simulink model "KERS_Gesamtmodell"  (Simulink 7.7)
settings: Solver=ode3  StartTime=0.0  StopTime=50.0  FixedStep=TiSample  RelTol=1e-3
model workspace: external: MAT-File ModelWorkspaceGesamtmodell.mat (data not in the file)
values from neighbouring files (symbols this model uses):
  ICnvrSyrmDqMax = 100    [ModelWorkspaceGesamtmodell.mat]
  SpdRtrMecIniVal = 2100    [ModelWorkspaceGesamtmodell.mat]
  SpdRtrMecMax = 2827    [ModelWorkspaceGesamtmodell.mat]
  SpdRtrMecMin = 1131    [ModelWorkspaceGesamtmodell.mat]
  TiSample = 2.5e-06    [ModelWorkspaceGesamtmodell.mat]
  UDcIniVal = 500    [ModelWorkspaceGesamtmodell.mat]
undefined symbols (not defined in the file or in its folder): CDc, CoeffFiltK, CoeffFiltP, CoeffFiltZ, DiscIntNeverNeededParam, JRtr, LSyrmCoilDq_d, LSyrmCoilDq_q, magnitude, NrOfPolePairs, RRepSyrmFeLoss, RSyrmCoilDq
libraries: KERS_SystemModel_lib x29, simulink x6
settings Model: MinMaxOverflowLogging=MinMaxAndOverflow  Creator=johannes.krettek  LastModifiedBy=johannes.krettek
settings DataIOCC: SaveOutput=off  InspectSignalLogs=on  SignalLoggingName=workingLog
settings DebuggingCC: SignalInfNanChecking=warning  UniqueDataStoreMsg=warning

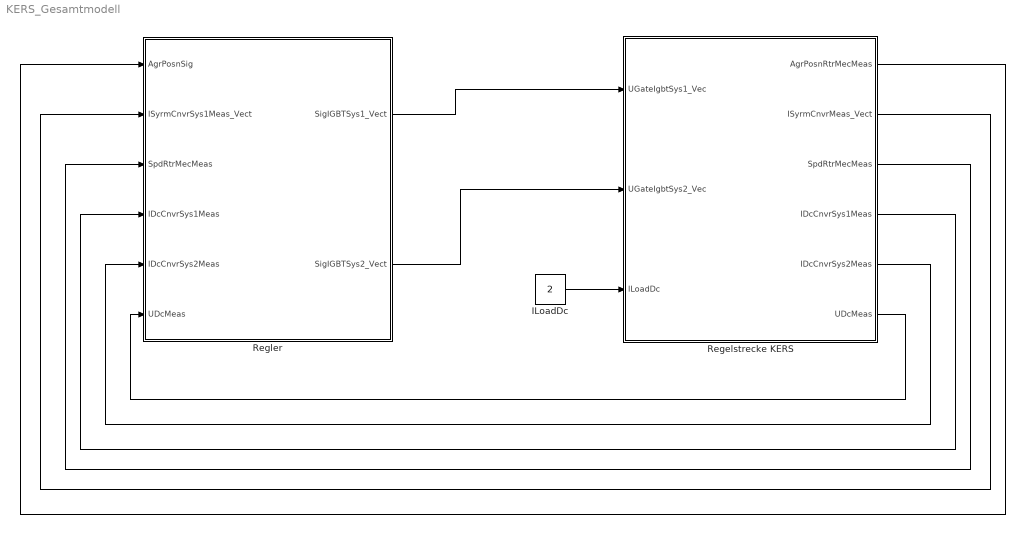
== system KERS_Gesamtmodell ==
  ILoadDc : Constant  Value=2
  Regelstrecke KERS : Subsystem
  Regler : Subsystem
  wires:
  Regler/1(SigIGBTSys1_Vect) -> Regelstrecke KERS/1(UGateIgbtSys1_Vec)
  Regelstrecke KERS/1(AgrPosnRtrMecMeas) -> Regler/1(AgrPosnSig)
  Regelstrecke KERS/2(ISyrmCnvrMeas_Vect) -> Regler/2(ISyrmCnvrSys1Meas_Vect)
  ILoadDc/1 -> Regelstrecke KERS/3(ILoadDc)
  Regler/2(SigIGBTSys2_Vect) -> Regelstrecke KERS/2(UGateIgbtSys2_Vec)
  Regelstrecke KERS/4(IDcCnvrSys1Meas) -> Regler/4(IDcCnvrSys1Meas)
  Regelstrecke KERS/5(IDcCnvrSys2Meas) -> Regler/5(IDcCnvrSys2Meas)
  Regelstrecke KERS/6(UDcMeas) -> Regler/6(UDcMeas)
  Regelstrecke KERS/3(SpdRtrMecMeas) -> Regler/3(SpdRtrMecMeas)

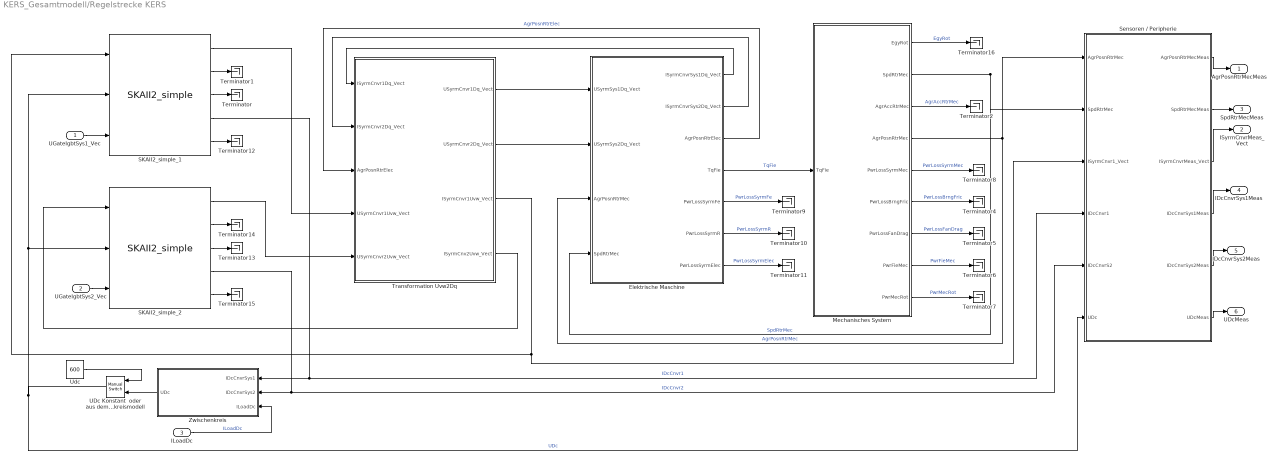
== system KERS_Gesamtmodell/Regelstrecke KERS ==
  UGateIgbtSys1_Vec : Inport  Interpolate=off
  UGateIgbtSys2_Vec : Inport  Port=2  Interpolate=off
  ILoadDc : Inport  Port=3  Interpolate=off
  Elektrische Maschine : Subsystem
  Mechanisches System : Subsystem
  SKAII2_simple_1 : KERS_SystemModel_lib/Leistungselektronik/SKAII2_simple  SystemSampleTime=-1
  SKAII2_simple_2 : KERS_SystemModel_lib/Leistungselektronik/SKAII2_simple  SystemSampleTime=-1
  Sensoren / Peripherie : Subsystem
  Terminator{,1..2,4..16} (16 alike) : Terminator
  Transformation Uvw2Dq : Subsystem
  UDc Konstant  oder aus dem Zwischenkreismodell : simulink/Signal Routing/Manual Switch  SystemSampleTime=-1  sw=0  action=0  varsize=off
  Udc : Constant  Value=600
  Zwischenkreis : Subsystem
  AgrPosnRtrMecMeas : Outport
  ISyrmCnvrMeas_Vect : Outport  Port=2
  SpdRtrMecMeas : Outport  Port=3
  IDcCnvrSys1Meas : Outport  Port=4
  IDcCnvrSys2Meas : Outport  Port=5
  UDcMeas : Outport  Port=6
  wires:
  Mechanisches System/2(SpdRtrMec) -> Elektrische Maschine/4(SpdRtrMec), Sensoren / Peripherie/2(SpdRtrMec)  "SpdRtrMec"
  Mechanisches System/4(AgrPosnRtrMec) -> Elektrische Maschine/3(AgrPosnRtrMec), Sensoren / Peripherie/1(AgrPosnRtrMec)  "AgrPosnRtrMec"
  Elektrische Maschine/4(TqFie) -> Mechanisches System/1(TqFie)  "TqFie"
  UGateIgbtSys1_Vec/1 -> SKAII2_simple_1/3
  Mechanisches System/1(EgyRot) -> Terminator16/1  "EgyRot"
  Mechanisches System/3(AgrAccRtrMec) -> Terminator2/1  "AgrAccRtrMec"
  Elektrische Maschine/5(PwrLossSyrmFe) -> Terminator9/1  "PwrLossSyrmFe"
  Elektrische Maschine/7(PwrLossSyrmElec) -> Terminator11/1  "PwrLossSyrmElec"
  Mechanisches System/6(PwrLossBrngFric) -> Terminator4/1  "PwrLossBrngFric"
  Mechanisches System/7(PwrLossFanDrag) -> Terminator5/1  "PwrLossFanDrag"
  Mechanisches System/9(PwrMecRot) -> Terminator7/1  "PwrMecRot"
  Mechanisches System/5(PwrLossSyrmMec) -> Terminator8/1  "PwrLossSyrmMec"
  Mechanisches System/8(PwrFieMec) -> Terminator6/1  "PwrFieMec"
  Elektrische Maschine/6(PwrLossSyrmR) -> Terminator10/1  "PwrLossSyrmR"
  SKAII2_simple_1/2 -> Terminator1/1
  SKAII2_simple_1/3 -> Terminator/1
  SKAII2_simple_1/5 -> Terminator12/1
  SKAII2_simple_2/2 -> Terminator14/1
  SKAII2_simple_2/3 -> Terminator13/1
  SKAII2_simple_2/5 -> Terminator15/1
  SKAII2_simple_2/4 -> Zwischenkreis/2(IDcCnvrSys2), Sensoren / Peripherie/5(IDcCnvrS2)  "IDcCnvr2"
  UGateIgbtSys2_Vec/1 -> SKAII2_simple_2/3
  Transformation Uvw2Dq/4(ISyrmCnv2Uvw_Vect) -> SKAII2_simple_2/1
  Transformation Uvw2Dq/3(ISyrmCnvr1Uvw_Vect) -> SKAII2_simple_1/1, Sensoren / Peripherie/3(ISyrmCnvr1_Vect)
  Elektrische Maschine/1(ISyrmCnvrSys1Dq_Vect) -> Transformation Uvw2Dq/1(ISyrmCnvr1Dq_Vect)
  Elektrische Maschine/2(ISyrmCnvrSys2Dq_Vect) -> Transformation Uvw2Dq/2(ISyrmCnvr2Dq_Vect)
  Elektrische Maschine/3(AgrPosnRtrElec) -> Transformation Uvw2Dq/3(AgrPosnRtrElec)  "AgrPosnRtrElec"
  Transformation Uvw2Dq/1(USyrmCnvr1Dq_Vect) -> Elektrische Maschine/1(USyrmSys1Dq_Vect)
  Transformation Uvw2Dq/2(USyrmCnvr2Dq_Vect) -> Elektrische Maschine/2(USyrmSys2Dq_Vect)
  SKAII2_simple_1/1 -> Transformation Uvw2Dq/4(USyrmCnvr1Uvw_Vect)
  SKAII2_simple_2/1 -> Transformation Uvw2Dq/5(USyrmCnvr2Uvw_Vect)
  SKAII2_simple_1/4 -> Zwischenkreis/1(IDcCnvrSys1), Sensoren / Peripherie/4(IDcCnvr1)  "IDcCnvr1"
  ILoadDc/1 -> Zwischenkreis/3(ILoadDc)  "ILoadDc"
  Udc/1 -> UDc Konstant  oder aus dem Zwischenkreismodell/1
  Zwischenkreis/1(UDc) -> UDc Konstant  oder aus dem Zwischenkreismodell/2
  UDc Konstant  oder aus dem Zwischenkreismodell/1 -> SKAII2_simple_2/2, SKAII2_simple_1/2, Sensoren / Peripherie/6(UDc)  "UDc"
  Sensoren / Peripherie/3(ISyrmCnvrMeas_Vect) -> ISyrmCnvrMeas_Vect/1
  Sensoren / Peripherie/4(IDcCnvrSys1Meas) -> IDcCnvrSys1Meas/1
  Sensoren / Peripherie/5(IDcCnvrSys2Meas) -> IDcCnvrSys2Meas/1
  Sensoren / Peripherie/1(AgrPosnRtrMecMeas) -> AgrPosnRtrMecMeas/1
  Sensoren / Peripherie/6(UDcMeas) -> UDcMeas/1
  Sensoren / Peripherie/2(SpdRtrMecMeas) -> SpdRtrMecMeas/1

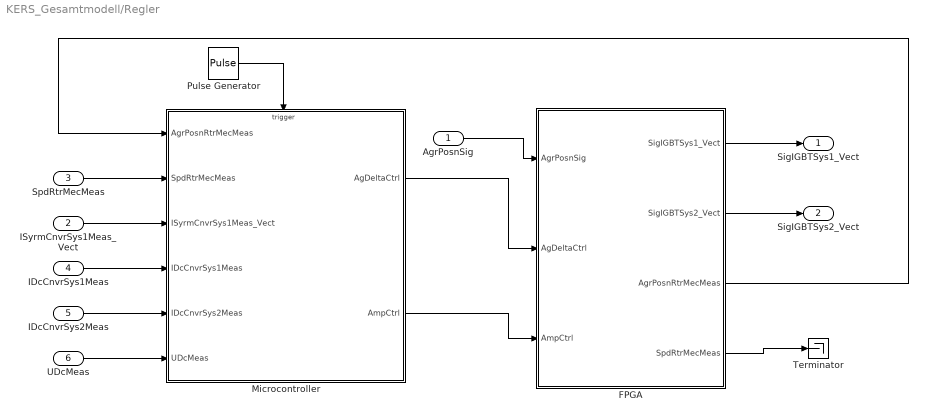
== system KERS_Gesamtmodell/Regler ==
  AgrPosnSig : Inport
  ISyrmCnvrSys1Meas_Vect : Inport  Port=2
  SpdRtrMecMeas : Inport  Port=3
  IDcCnvrSys1Meas : Inport  Port=4
  IDcCnvrSys2Meas : Inport  Port=5
  UDcMeas : Inport  Port=6
  FPGA : Subsystem
  Microcontroller : Subsystem
  Pulse Generator : DiscretePulseGenerator  PulseType=Time based  Period=TiSample*10  PulseWidth=50
  Terminator : Terminator
  SigIGBTSys1_Vect : Outport
  SigIGBTSys2_Vect : Outport  Port=2
  wires:
  FPGA/1(SigIGBTSys1_Vect) -> SigIGBTSys1_Vect/1
  FPGA/2(SigIGBTSys2_Vect) -> SigIGBTSys2_Vect/1
  Microcontroller/1(AgDeltaCtrl) -> FPGA/2(AgDeltaCtrl)
  Microcontroller/2(AmpCtrl) -> FPGA/3(AmpCtrl)
  AgrPosnSig/1 -> FPGA/1(AgrPosnSig)
  FPGA/3(AgrPosnRtrMecMeas) -> Microcontroller/1(AgrPosnRtrMecMeas)
  ISyrmCnvrSys1Meas_Vect/1 -> Microcontroller/3(ISyrmCnvrSys1Meas_Vect)
  IDcCnvrSys1Meas/1 -> Microcontroller/4(IDcCnvrSys1Meas)
  IDcCnvrSys2Meas/1 -> Microcontroller/5(IDcCnvrSys2Meas)
  UDcMeas/1 -> Microcontroller/6(UDcMeas)
  Pulse Generator/1 -> Microcontroller/Trigger
  SpdRtrMecMeas/1 -> Microcontroller/2(SpdRtrMecMeas)
  FPGA/4(SpdRtrMecMeas) -> Terminator/1

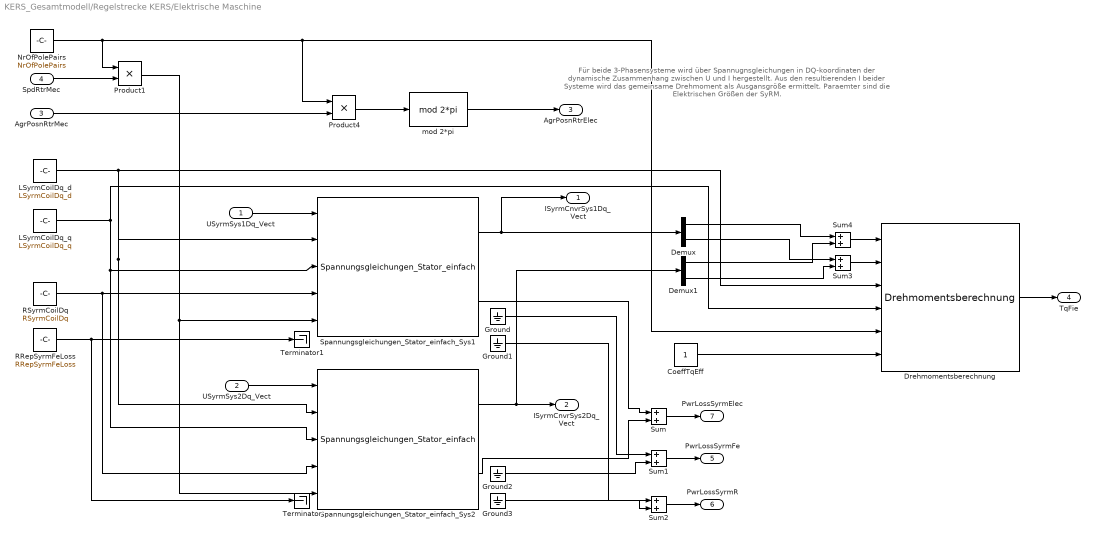
== system KERS_Gesamtmodell/Regelstrecke KERS/Elektrische Maschine ==
  note: Für beide 3-Phasensysteme wird über Spannugnsgleichungen in
      | DQ-koordinaten der dynamische Zusammenhang zwischen U und I
      | hergestellt. Aus den resultierenden I beider Systeme wird das
      | gemeinsame Drehmoment als Ausgansgröße ermittelt.
      | Paraemter sind die Elektrischen Größen der SyRM.
  USyrmSys1Dq_Vect : Inport
  USyrmSys2Dq_Vect : Inport  Port=2
  AgrPosnRtrMec : Inport  Port=3
  SpdRtrMec : Inport  Port=4
  CoeffTqEff : Constant  OutMin=0
  Demux : Demux  Outputs=2
  Demux1 : Demux  Outputs=2
  Drehmomentsberechnung : KERS_SystemModel_lib/Module Stator-Komponenten/Drehmomentsberechnung  SystemSampleTime=-1
  Ground{,1..3} (4 alike) : Ground
  LSyrmCoilDq_d : Constant  Value=LSyrmCoilDq_d  OutMin=0
  LSyrmCoilDq_q : Constant  Value=LSyrmCoilDq_q  OutMin=0
  NrOfPolePairs : Constant  Value=NrOfPolePairs
  Product1 : Product  RndMeth=Zero
  Product4 : Product  RndMeth=Zero
  RRepSyrmFeLoss : Constant  Value=RRepSyrmFeLoss  OutMin=0
  RSyrmCoilDq : Constant  Value=RSyrmCoilDq  OutMin=0
  Spannungsgleichungen_Stator_einfach_Sys1 : KERS_SystemModel_lib/Module Stator-Komponenten/Spannungsgleichungen_Stator_einfach  SystemSampleTime=-1
  Spannungsgleichungen_Stator_einfach_Sys2 : KERS_SystemModel_lib/Module Stator-Komponenten/Spannungsgleichungen_Stator_einfach  SystemSampleTime=-1
  Sum{,1..4} (5 alike) : Sum
  Terminator : Terminator
  Terminator1 : Terminator
  mod 2*pi : KERS_SystemModel_lib/Transformationen/mod 2*pi  SystemSampleTime=-1  tau=2*pi
  ISyrmCnvrSys1Dq_Vect : Outport
  ISyrmCnvrSys2Dq_Vect : Outport  Port=2
  AgrPosnRtrElec : Outport  Port=3
  TqFie : Outport  Port=4
  PwrLossSyrmFe : Outport  Port=5
  PwrLossSyrmR : Outport  Port=6
  PwrLossSyrmElec : Outport  Port=7
  wires:
  Drehmomentsberechnung/1 -> TqFie/1
  LSyrmCoilDq_d/1 -> Drehmomentsberechnung/3, Spannungsgleichungen_Stator_einfach_Sys2/2, Spannungsgleichungen_Stator_einfach_Sys1/2
  LSyrmCoilDq_q/1 -> Drehmomentsberechnung/4, Spannungsgleichungen_Stator_einfach_Sys1/3, Spannungsgleichungen_Stator_einfach_Sys2/3
  NrOfPolePairs/1 -> Product4/1, Drehmomentsberechnung/5, Product1/1
  Product4/1 -> mod 2*pi/1
  Product1/1 -> Spannungsgleichungen_Stator_einfach_Sys2/5, Spannungsgleichungen_Stator_einfach_Sys1/5
  Spannungsgleichungen_Stator_einfach_Sys1/1 -> ISyrmCnvrSys1Dq_Vect/1, Demux/1
  RSyrmCoilDq/1 -> Spannungsgleichungen_Stator_einfach_Sys1/4, Spannungsgleichungen_Stator_einfach_Sys2/4
  AgrPosnRtrMec/1 -> Product4/2
  RRepSyrmFeLoss/1 -> Terminator/1, Terminator1/1
  CoeffTqEff/1 -> Drehmomentsberechnung/6
  mod 2*pi/1 -> AgrPosnRtrElec/1
  Spannungsgleichungen_Stator_einfach_Sys2/1 -> ISyrmCnvrSys2Dq_Vect/1, Demux1/1
  USyrmSys2Dq_Vect/1 -> Spannungsgleichungen_Stator_einfach_Sys2/1
  Sum/1 -> PwrLossSyrmElec/1
  Sum1/1 -> PwrLossSyrmFe/1
  Sum2/1 -> PwrLossSyrmR/1
  Spannungsgleichungen_Stator_einfach_Sys2/2 -> Sum/2
  Ground/1 -> Sum1/1
  Ground2/1 -> Sum1/2
  Ground1/1 -> Sum2/1
  Ground3/1 -> Sum2/2
  Demux/1 -> Sum4/1
  Demux1/1 -> Sum4/2
  Demux/2 -> Sum3/1
  Demux1/2 -> Sum3/2
  Sum4/1 -> Drehmomentsberechnung/1
  Sum3/1 -> Drehmomentsberechnung/2
  Spannungsgleichungen_Stator_einfach_Sys1/2 -> Sum/1
  USyrmSys1Dq_Vect/1 -> Spannungsgleichungen_Stator_einfach_Sys1/1
  SpdRtrMec/1 -> Product1/2

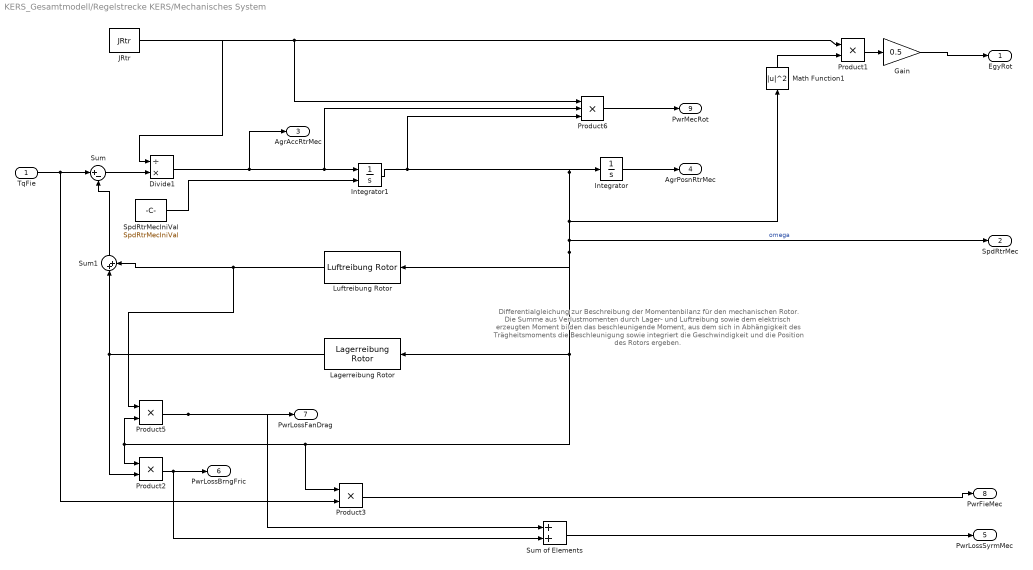
== system KERS_Gesamtmodell/Regelstrecke KERS/Mechanisches System ==
  note: Differentialgleichung zur Beschreibung der Momentenbilanz für den mechanischen Rotor.
      | Die Summe aus Verlustmomenten durch Lager- und Luftreibung sowie dem elektrisch erzeugten
      | Moment bilden das beschleunigende Moment, aus dem sich in Abhängigkeit des Trägheitsmoments
      | die Beschleunigung sowie integriert die Geschwindigkeit und die Position des Rotors ergeben.
  TqFie : Inport
  Divide1 : Product  Inputs=/*
  Gain : Gain  Gain=0.5
  Integrator : Integrator
  Integrator1 : Integrator  InitialConditionSource=external
  JRtr : Constant  Value=JRtr
  Lagerreibung Rotor : KERS_SystemModel_lib/Module Rotor-Komponenten/Lagerreibung Rotor  SystemSampleTime=-1
  Luftreibung Rotor : KERS_SystemModel_lib/Module Rotor-Komponenten/Luftreibung Rotor  SystemSampleTime=-1
  Math Function1 : Math  Operator=magnitude^2  SaturateOnIntegerOverflow=on
  Product{1..3,5} (4 alike) : Product  RndMeth=Zero
  Product6 : Product  Inputs=3  RndMeth=Zero
  SpdRtrMecIniVal : Constant  Value=SpdRtrMecIniVal
  Sum : Sum  Inputs=|+-
  Sum of Elements : Sum
  Sum1 : Sum  Inputs=|++
  EgyRot : Outport
  SpdRtrMec : Outport  Port=2
  AgrAccRtrMec : Outport  Port=3
  AgrPosnRtrMec : Outport  Port=4
  PwrLossSyrmMec : Outport  Port=5
  PwrLossBrngFric : Outport  Port=6
  PwrLossFanDrag : Outport  Port=7
  PwrFieMec : Outport  Port=8
  PwrMecRot : Outport  Port=9
  wires:
  TqFie/1 -> Sum/1, Product3/2
  Sum1/1 -> Sum/2
  Integrator/1 -> AgrPosnRtrMec/1
  Luftreibung Rotor/1 -> Sum1/2, Product5/1
  Lagerreibung Rotor/1 -> Sum1/1, Product2/2
  JRtr/1 -> Divide1/1, Product1/1, Product6/1
  Product1/1 -> Gain/1
  Product2/1 -> PwrLossBrngFric/1, Sum of Elements/2
  Product5/1 -> PwrLossFanDrag/1, Sum of Elements/1
  Product3/1 -> PwrFieMec/1
  Integrator1/1 -> Product5/2, Product2/1, Product3/1, Lagerreibung Rotor/1, Luftreibung Rotor/1, SpdRtrMec/1, Math Function1/1, Integrator/1, Product6/3  "omega"
  Divide1/1 -> AgrAccRtrMec/1, Product6/2, Integrator1/1
  Sum/1 -> Divide1/2
  SpdRtrMecIniVal/1 -> Integrator1/2
  Gain/1 -> EgyRot/1
  Product6/1 -> PwrMecRot/1
  Sum of Elements/1 -> PwrLossSyrmMec/1
  Math Function1/1 -> Product1/2

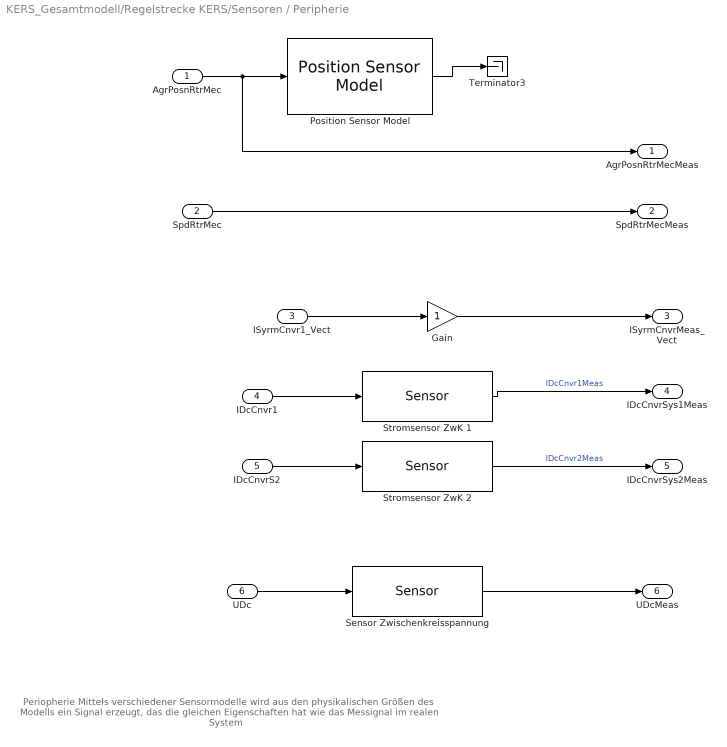
== system KERS_Gesamtmodell/Regelstrecke KERS/Sensoren / Peripherie ==
  note: Periopherie
      | Mittels verschiedener Sensormodelle wird aus den physikalischen Größen
      | des Modells ein Signal erzeugt, das die gleichen Eigenschaften hat wie
      | das Messignal im realen System
  AgrPosnRtrMec : Inport
  SpdRtrMec : Inport  Port=2
  ISyrmCnvr1_Vect : Inport  Port=3
  IDcCnvr1 : Inport  Port=4
  IDcCnvrS2 : Inport  Port=5
  UDc : Inport  Port=6
  Gain : Gain
  Position Sensor Model : KERS_SystemModel_lib/Peripheral Modules/Position Sensor Model  SystemSampleTime=-1  PosnSens1Offset=0.1  PosnSens2Offset=pi  PosnSensWidth=0.2
  Sensor Zwischenkreisspannung : KERS_SystemModel_lib/Peripheral Modules/Sensor  SystemSampleTime=-1
  Stromsensor ZwK 1 : KERS_SystemModel_lib/Peripheral Modules/Sensor  SystemSampleTime=-1
      link override Transport Delay: DelayTime=TiSample
  Stromsensor ZwK 2 : KERS_SystemModel_lib/Peripheral Modules/Sensor  SystemSampleTime=-1
      link override Transport Delay: DelayTime=TiSample
  Terminator3 : Terminator
  AgrPosnRtrMecMeas : Outport
  SpdRtrMecMeas : Outport  Port=2
  ISyrmCnvrMeas_Vect : Outport  Port=3
  IDcCnvrSys1Meas : Outport  Port=4
  IDcCnvrSys2Meas : Outport  Port=5
  UDcMeas : Outport  Port=6
  wires:
  Stromsensor ZwK 1/1 -> IDcCnvrSys1Meas/1  "IDcCnvr1Meas"
  Stromsensor ZwK 2/1 -> IDcCnvrSys2Meas/1  "IDcCnvr2Meas"
  Sensor Zwischenkreisspannung/1 -> UDcMeas/1
  ISyrmCnvr1_Vect/1 -> Gain/1
  AgrPosnRtrMec/1 -> Position Sensor Model/1, AgrPosnRtrMecMeas/1
  UDc/1 -> Sensor Zwischenkreisspannung/1
  IDcCnvr1/1 -> Stromsensor ZwK 1/1
  IDcCnvrS2/1 -> Stromsensor ZwK 2/1
  SpdRtrMec/1 -> SpdRtrMecMeas/1
  Gain/1 -> ISyrmCnvrMeas_Vect/1
  Position Sensor Model/1 -> Terminator3/1

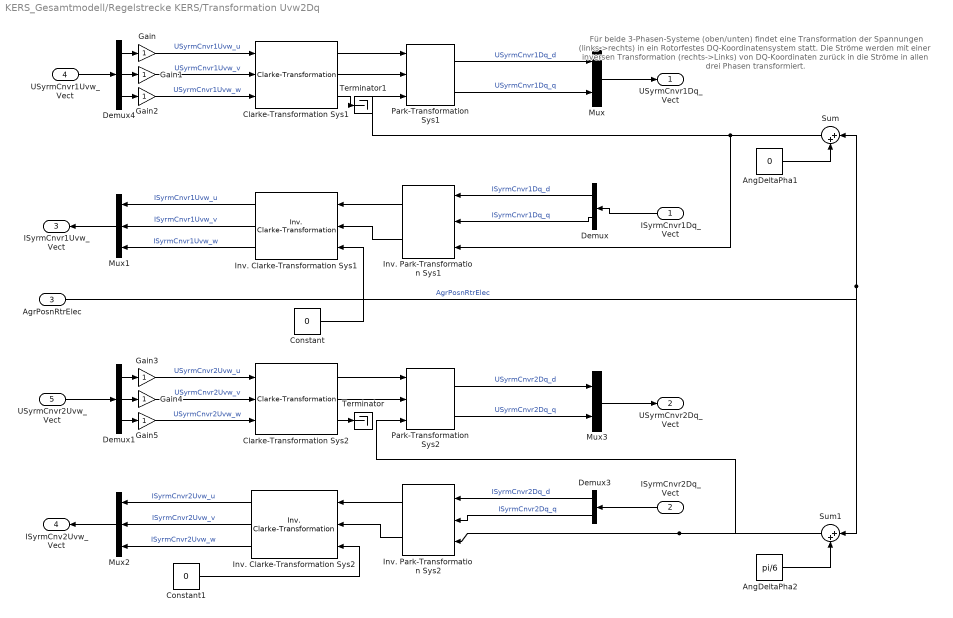
== system KERS_Gesamtmodell/Regelstrecke KERS/Transformation Uvw2Dq ==
  note: Für beide 3-Phasen-Systeme (oben/unten) findet eine Transformation
      | der Spannungen (links->rechts) in ein Rotorfestes DQ-Koordinatensystem statt.
      | Die Ströme werden mit einer inversen Transformation (rechts->Links)
      | von DQ-Koordinaten zurück in die Ströme in allen drei Phasen transformiert.
  ISyrmCnvr1Dq_Vect : Inport
  ISyrmCnvr2Dq_Vect : Inport  Port=2
  AgrPosnRtrElec : Inport  Port=3
  USyrmCnvr1Uvw_Vect : Inport  Port=4
  USyrmCnvr2Uvw_Vect : Inport  Port=5
  AngDeltaPha1 : Constant  Value=0
  AngDeltaPha2 : Constant  Value=pi/6
  Clarke-Transformation Sys1 : KERS_SystemModel_lib/Transformationen/Clarke-Transformation  SystemSampleTime=-1
  Clarke-Transformation Sys2 : KERS_SystemModel_lib/Transformationen/Clarke-Transformation  SystemSampleTime=-1
  Constant : Constant  Value=0
  Constant1 : Constant  Value=0
  Demux : Demux  Outputs=2
  Demux1 : Demux  Outputs=3
  Demux3 : Demux  Outputs=2
  Demux4 : Demux  Outputs=3
  Gain{,1..5} (6 alike) : Gain
  Inv. Clarke-Transformation Sys1 : KERS_SystemModel_lib/Transformationen/Inv. Clarke-Transformation  SystemSampleTime=-1
  Inv. Clarke-Transformation Sys2 : KERS_SystemModel_lib/Transformationen/Inv. Clarke-Transformation  SystemSampleTime=-1
  Inv. Park-Transformation Sys1 : KERS_SystemModel_lib/Transformationen/Inv. Park-Transformation  SystemSampleTime=-1
  Inv. Park-Transformation Sys2 : KERS_SystemModel_lib/Transformationen/Inv. Park-Transformation  SystemSampleTime=-1
  Mux : Mux  Inputs=2
  Mux1 : Mux  Inputs=3
  Mux2 : Mux  Inputs=3
  Mux3 : Mux  Inputs=2
  Park-Transformation Sys1 : KERS_SystemModel_lib/Transformationen/Park-Transformation  SystemSampleTime=-1
  Park-Transformation Sys2 : KERS_SystemModel_lib/Transformationen/Park-Transformation  SystemSampleTime=-1
  Sum : Sum  Inputs=|++
  Sum1 : Sum  Inputs=|++
  Terminator : Terminator
  Terminator1 : Terminator
  USyrmCnvr1Dq_Vect : Outport
  USyrmCnvr2Dq_Vect : Outport  Port=2
  ISyrmCnvr1Uvw_Vect : Outport  Port=3
  ISyrmCnv2Uvw_Vect : Outport  Port=4
  wires:
  Inv. Park-Transformation Sys1/1 -> Inv. Clarke-Transformation Sys1/1
  Inv. Park-Transformation Sys1/2 -> Inv. Clarke-Transformation Sys1/2
  Demux/1 -> Inv. Park-Transformation Sys1/1  "ISyrmCnvr1Dq_d"
  Demux/2 -> Inv. Park-Transformation Sys1/2  "ISyrmCnvr1Dq_q"
  Park-Transformation Sys1/1 -> Mux/1  "USyrmCnvr1Dq_d"
  Park-Transformation Sys1/2 -> Mux/2  "USyrmCnvr1Dq_q"
  Inv. Clarke-Transformation Sys1/1 -> Mux1/1  "ISyrmCnvr1Uvw_u"
  Inv. Clarke-Transformation Sys1/2 -> Mux1/2  "ISyrmCnvr1Uvw_v"
  Inv. Clarke-Transformation Sys1/3 -> Mux1/3  "ISyrmCnvr1Uvw_w"
  ISyrmCnvr1Dq_Vect/1 -> Demux/1
  Mux/1 -> USyrmCnvr1Dq_Vect/1
  Gain/1 -> Clarke-Transformation Sys1/1  "USyrmCnvr1Uvw_u"
  Gain1/1 -> Clarke-Transformation Sys1/2  "USyrmCnvr1Uvw_v"
  Gain2/1 -> Clarke-Transformation Sys1/3  "USyrmCnvr1Uvw_w"
  Gain3/1 -> Clarke-Transformation Sys2/1  "USyrmCnvr2Uvw_u"
  Gain4/1 -> Clarke-Transformation Sys2/2  "USyrmCnvr2Uvw_v"
  Gain5/1 -> Clarke-Transformation Sys2/3  "USyrmCnvr2Uvw_w"
  Clarke-Transformation Sys1/1 -> Park-Transformation Sys1/1
  Clarke-Transformation Sys1/2 -> Park-Transformation Sys1/2
  AgrPosnRtrElec/1 -> Sum/1, Sum1/1  "AgrPosnRtrElec"
  AngDeltaPha1/1 -> Sum/2
  Sum/1 -> Inv. Park-Transformation Sys1/3, Park-Transformation Sys1/3
  AngDeltaPha2/1 -> Sum1/2
  Clarke-Transformation Sys2/1 -> Park-Transformation Sys2/1
  Clarke-Transformation Sys2/2 -> Park-Transformation Sys2/2
  Demux3/1 -> Inv. Park-Transformation Sys2/1  "ISyrmCnvr2Dq_d"
  Demux3/2 -> Inv. Park-Transformation Sys2/2  "ISyrmCnvr2Dq_q"
  Sum1/1 -> Inv. Park-Transformation Sys2/3, Park-Transformation Sys2/3
  Inv. Park-Transformation Sys2/1 -> Inv. Clarke-Transformation Sys2/1
  Inv. Park-Transformation Sys2/2 -> Inv. Clarke-Transformation Sys2/2
  Inv. Clarke-Transformation Sys2/1 -> Mux2/1  "ISyrmCnvr2Uvw_u"
  Inv. Clarke-Transformation Sys2/2 -> Mux2/2  "ISyrmCnvr2Uvw_v"
  Inv. Clarke-Transformation Sys2/3 -> Mux2/3  "ISyrmCnvr2Uvw_w"
  Park-Transformation Sys2/1 -> Mux3/1  "USyrmCnvr2Dq_d"
  Park-Transformation Sys2/2 -> Mux3/2  "USyrmCnvr2Dq_q"
  Mux3/1 -> USyrmCnvr2Dq_Vect/1
  ISyrmCnvr2Dq_Vect/1 -> Demux3/1
  Mux1/1 -> ISyrmCnvr1Uvw_Vect/1
  Mux2/1 -> ISyrmCnv2Uvw_Vect/1
  Demux4/1 -> Gain/1
  Demux4/2 -> Gain1/1
  Demux4/3 -> Gain2/1
  USyrmCnvr1Uvw_Vect/1 -> Demux4/1
  Demux1/1 -> Gain3/1
  Demux1/2 -> Gain4/1
  Demux1/3 -> Gain5/1
  USyrmCnvr2Uvw_Vect/1 -> Demux1/1
  Constant/1 -> Inv. Clarke-Transformation Sys1/3
  Constant1/1 -> Inv. Clarke-Transformation Sys2/3
  Clarke-Transformation Sys2/3 -> Terminator/1
  Clarke-Transformation Sys1/3 -> Terminator1/1

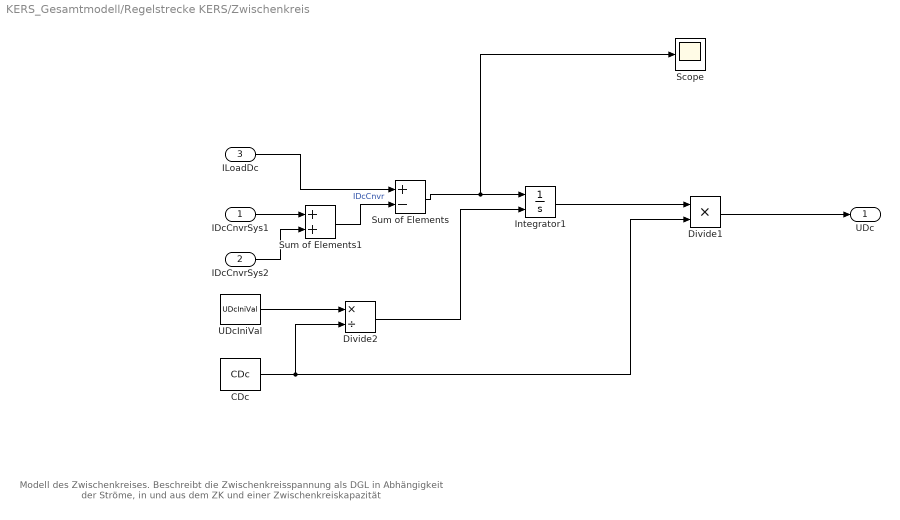
== system KERS_Gesamtmodell/Regelstrecke KERS/Zwischenkreis ==
  note: Modell des Zwischenkreises. Beschreibt die Zwischenkreisspannung als
      | DGL in Abhängigkeit der Ströme, in und aus dem ZK und einer Zwischenkreiskapazität
  IDcCnvrSys1 : Inport
  IDcCnvrSys2 : Inport  Port=2
  ILoadDc : Inport  Port=3
  CDc : Constant  Value=CDc
  Divide1 : Product  Inputs=**
  Divide2 : Product  Inputs=*/
  Integrator1 : Integrator  InitialConditionSource=external
  Scope : Scope
  Sum of Elements : Sum  Inputs=+-
  Sum of Elements1 : Sum
  UDcIniVal : Constant  Value=UDcIniVal
  UDc : Outport
  wires:
  ILoadDc/1 -> Sum of Elements/1
  Sum of Elements/1 -> Integrator1/1, Scope/1
  Integrator1/1 -> Divide1/1
  CDc/1 -> Divide1/2, Divide2/2
  UDcIniVal/1 -> Divide2/1
  Divide2/1 -> Integrator1/2
  Divide1/1 -> UDc/1
  Sum of Elements1/1 -> Sum of Elements/2  "IDcCnvr"
  IDcCnvrSys1/1 -> Sum of Elements1/1
  IDcCnvrSys2/1 -> Sum of Elements1/2

== system KERS_Gesamtmodell/Regler/FPGA ==
  note: Aktuell: Erzeugung des Ansteuersignals für die LEs aus Amplitude und Phase
      | des ideal vorgegebenen Spannungszeigers durch eine Sinus-Dreiecks-Modulation
      | Geplant: Auswertung der Positionssensoren durch eine PLL, Erweiterung der
      | Ansteuerung um einen Anlauf mit PWM
  AgrPosnSig : Inport
  AgDeltaCtrl : Inport  Port=2
  AmpCtrl : Inport  Port=3
  Ansteuerung LE : Subsystem
  Ground : Ground
  Polpaarzahl : Gain  Gain=NrOfPolePairs
  mod 2*pi : KERS_SystemModel_lib/Transformationen/mod 2*pi  SystemSampleTime=-1  tau=2*pi
  SigIGBTSys1_Vect : Outport
  SigIGBTSys2_Vect : Outport  Port=2
  AgrPosnRtrMecMeas : Outport  Port=3
  SpdRtrMecMeas : Outport  Port=4
  wires:
  Ansteuerung LE/1(SigIGBTSys1_Vect) -> SigIGBTSys1_Vect/1
  Ansteuerung LE/2(SigIGBTSys2_Vect) -> SigIGBTSys2_Vect/1
  AmpCtrl/1 -> Ansteuerung LE/3(AmpCtrl)
  AgDeltaCtrl/1 -> Ansteuerung LE/2(AgDeltaCtrl)
  AgrPosnSig/1 -> AgrPosnRtrMecMeas/1, Polpaarzahl/1
  mod 2*pi/1 -> Ansteuerung LE/1(AgrPosnEl)
  Polpaarzahl/1 -> mod 2*pi/1
  Ground/1 -> SpdRtrMecMeas/1

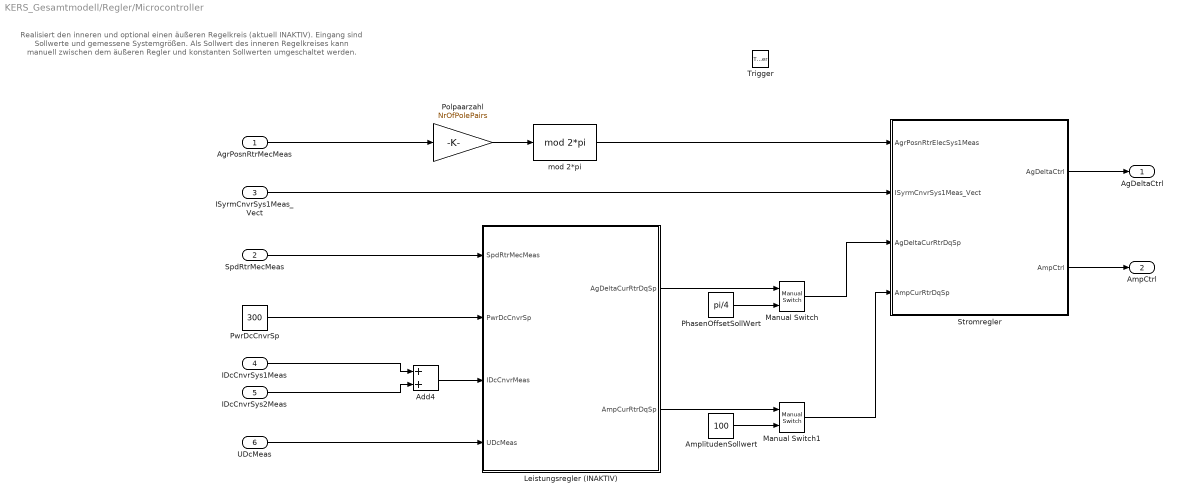
== system KERS_Gesamtmodell/Regler/Microcontroller ==
  note: Realisiert den inneren und optional einen äußeren Regelkreis (aktuell INAKTIV).
      | Eingang sind Sollwerte und gemessene Systemgrößen. Als Sollwert des inneren
      | Regelkreises kann manuell zwischen dem äußeren Regler und konstanten
      | Sollwerten umgeschaltet werden.
  AgrPosnRtrMecMeas : Inport
  SpdRtrMecMeas : Inport  Port=2
  ISyrmCnvrSys1Meas_Vect : Inport  Port=3
  IDcCnvrSys1Meas : Inport  Port=4
  IDcCnvrSys2Meas : Inport  Port=5
  UDcMeas : Inport  Port=6
  Trigger : TriggerPort
  Add4 : Sum
  AmplitudenSollwert : Constant  Value=100  SampleTime=-1
  Leistungsregler (INAKTIV) : Subsystem
  Manual Switch : simulink/Signal Routing/Manual Switch  SystemSampleTime=-1  sw=0  action=0  varsize=off
  Manual Switch1 : simulink/Signal Routing/Manual Switch  SystemSampleTime=-1  sw=0  action=0  varsize=off
  PhasenOffsetSollWert : Constant  Value=pi/4
  Polpaarzahl : Gain  Gain=NrOfPolePairs
  PwrDcCnvrSp : Constant  Value=300  SampleTime=-1
  Stromregler : Subsystem
  mod 2*pi : KERS_SystemModel_lib/Transformationen/mod 2*pi  SystemSampleTime=-1  tau=2*pi
  AgDeltaCtrl : Outport
  AmpCtrl : Outport  Port=2
  wires:
  ISyrmCnvrSys1Meas_Vect/1 -> Stromregler/2(ISyrmCnvrSys1Meas_Vect)
  AgrPosnRtrMecMeas/1 -> Polpaarzahl/1
  Stromregler/1(AgDeltaCtrl) -> AgDeltaCtrl/1
  Stromregler/2(AmpCtrl) -> AmpCtrl/1
  Manual Switch/1 -> Stromregler/3(AgDeltaCurRtrDqSp)
  PhasenOffsetSollWert/1 -> Manual Switch/2
  Manual Switch1/1 -> Stromregler/4(AmpCurRtrDqSp)
  AmplitudenSollwert/1 -> Manual Switch1/2
  PwrDcCnvrSp/1 -> Leistungsregler (INAKTIV)/2(PwrDcCnvrSp)
  Leistungsregler (INAKTIV)/1(AgDeltaCurRtrDqSp) -> Manual Switch/1
  Leistungsregler (INAKTIV)/2(AmpCurRtrDqSp) -> Manual Switch1/1
  IDcCnvrSys1Meas/1 -> Add4/1
  IDcCnvrSys2Meas/1 -> Add4/2
  SpdRtrMecMeas/1 -> Leistungsregler (INAKTIV)/1(SpdRtrMecMeas)
  UDcMeas/1 -> Leistungsregler (INAKTIV)/4(UDcMeas)
  Add4/1 -> Leistungsregler (INAKTIV)/3(IDcCnvrMeas)
  Polpaarzahl/1 -> mod 2*pi/1
  mod 2*pi/1 -> Stromregler/1(AgrPosnRtrElecSys1Meas)

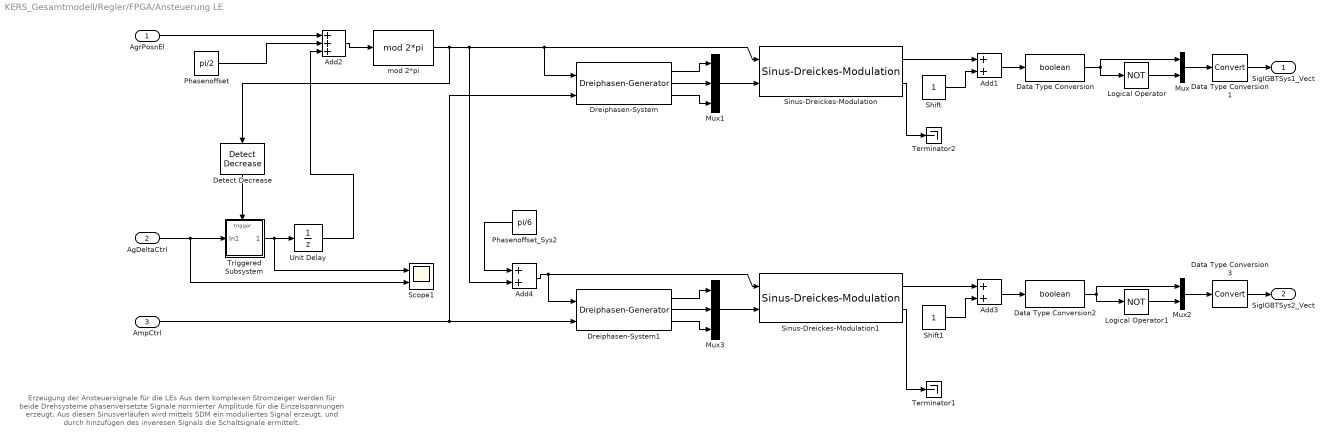
== system KERS_Gesamtmodell/Regler/FPGA/Ansteuerung LE ==
  note: Erzeugung der Ansteuersignale für die LEs
      | Aus dem komplexen Stromzeiger werden für beide Drehsysteme
      | phasenversetzte Signale normierter Amplitude für die Einzelspannungen erzeugt.
      | Aus diesen Sinusverläufen wird mittels SDM ein moduliertes Signal erzeugt,
      | und durch hinzufügen des inveresen Signals die Schaltsignale ermittelt.
  AgrPosnEl : Inport
  AgDeltaCtrl : Inport  Port=2
  AmpCtrl : Inport  Port=3
  Add1 : Sum
  Add2 : Sum  Inputs=+++
  Add3 : Sum
  Add4 : Sum
  Data Type Conversion : DataTypeConversion  OutDataTypeStr=boolean
  Data Type Conversion1 : DataTypeConversion
  Data Type Conversion2 : DataTypeConversion  OutDataTypeStr=boolean
  Data Type Conversion3 : DataTypeConversion
  Detect Decrease : simulink/Logic and Bit Operations/Detect Decrease  SystemSampleTime=-1  vinit=0.0
  Dreiphasen-System : KERS_SystemModel_lib/Leistungselektronik/Dreiphasen-Generator  SystemSampleTime=-1
  Dreiphasen-System1 : KERS_SystemModel_lib/Leistungselektronik/Dreiphasen-Generator  SystemSampleTime=-1
  Logical Operator : Logic  Operator=NOT  AllPortsSameDT=off  OutDataTypeStr=boolean
  Logical Operator1 : Logic  Operator=NOT  AllPortsSameDT=off  OutDataTypeStr=boolean
  Mux : Mux  Inputs=2
  Mux1 : Mux  Inputs=3
  Mux2 : Mux  Inputs=2
  Mux3 : Mux  Inputs=3
  Phasenoffset : Constant  Value=pi/2
  Phasenoffset_Sys2 : Constant  Value=pi/6
  Scope1 : Scope  NumInputPorts=2
      settings: YMin=0~-5  YMax=6.5~5
  Shift : Constant
  Shift1 : Constant
  Sinus-Dreickes-Modulation : KERS_SystemModel_lib/Leistungselektronik/Sinus-Dreickes-Modulation  SystemSampleTime=-1
  Sinus-Dreickes-Modulation1 : KERS_SystemModel_lib/Leistungselektronik/Sinus-Dreickes-Modulation  SystemSampleTime=-1
  Terminator1 : Terminator
  Terminator2 : Terminator
  Triggered Subsystem : Subsystem  TreatAsAtomicUnit=on
  Unit Delay : UnitDelay  SampleTime=-1
  mod 2*pi : KERS_SystemModel_lib/Transformationen/mod 2*pi  SystemSampleTime=-1  tau=2*pi
  SigIGBTSys1_Vect : Outport
  SigIGBTSys2_Vect : Outport  Port=2
  wires:
  AgrPosnEl/1 -> Add2/1
  Dreiphasen-System/1 -> Mux1/1
  Mux1/1 -> Sinus-Dreickes-Modulation/2
  Data Type Conversion/1 -> Logical Operator/1, Mux/1
  Logical Operator/1 -> Mux/2
  Mux/1 -> Data Type Conversion1/1
  Data Type Conversion1/1 -> SigIGBTSys1_Vect/1
  Sinus-Dreickes-Modulation/1 -> Add1/1
  Add1/1 -> Data Type Conversion/1
  Shift/1 -> Add1/2
  Dreiphasen-System/2 -> Mux1/2
  Dreiphasen-System/3 -> Mux1/3
  AgDeltaCtrl/1 -> Triggered Subsystem/1(In1), Scope1/2
  Add2/1 -> mod 2*pi/1
  Triggered Subsystem/1(Out1) -> Unit Delay/1, Scope1/1
  Detect Decrease/1 -> Triggered Subsystem/Trigger
  mod 2*pi/1 -> Sinus-Dreickes-Modulation/1, Dreiphasen-System/1, Add4/2, Detect Decrease/1
  Unit Delay/1 -> Add2/3
  Dreiphasen-System1/1 -> Mux3/1
  Mux3/1 -> Sinus-Dreickes-Modulation1/2
  Data Type Conversion2/1 -> Logical Operator1/1, Mux2/1
  Logical Operator1/1 -> Mux2/2
  Mux2/1 -> Data Type Conversion3/1
  Data Type Conversion3/1 -> SigIGBTSys2_Vect/1
  Sinus-Dreickes-Modulation1/1 -> Add3/1
  Add3/1 -> Data Type Conversion2/1
  Shift1/1 -> Add3/2
  Dreiphasen-System1/2 -> Mux3/2
  Dreiphasen-System1/3 -> Mux3/3
  Add4/1 -> Dreiphasen-System1/1, Sinus-Dreickes-Modulation1/1
  Phasenoffset_Sys2/1 -> Add4/1
  Phasenoffset/1 -> Add2/2
  AmpCtrl/1 -> Dreiphasen-System1/2, Dreiphasen-System/2
  Sinus-Dreickes-Modulation1/2 -> Terminator1/1
  Sinus-Dreickes-Modulation/2 -> Terminator2/1

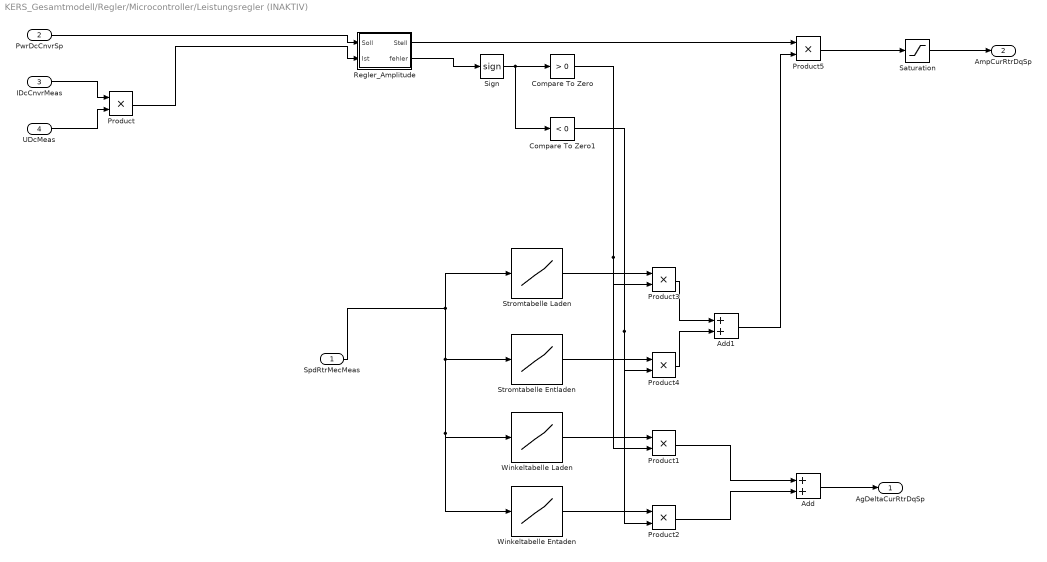
== system KERS_Gesamtmodell/Regler/Microcontroller/Leistungsregler (INAKTIV) ==
  SpdRtrMecMeas : Inport
  PwrDcCnvrSp : Inport  Port=2
  IDcCnvrMeas : Inport  Port=3
  UDcMeas : Inport  Port=4
  Add : Sum
  Add1 : Sum
  Compare To Zero : simulink/Logic and Bit Operations/Compare To Zero  SystemSampleTime=-1  relop=>  LogicOutDataTypeMode=uint8
  Compare To Zero1 : simulink/Logic and Bit Operations/Compare To Zero  SystemSampleTime=-1  relop=<  LogicOutDataTypeMode=uint8
  Product{,1..5} (6 alike) : Product  RndMeth=Zero
  Regler_Amplitude : Subsystem
  Saturation : Saturate  UpperLimit=ICnvrSyrmDqMax  LowerLimit=-1*ICnvrSyrmDqMax
  Sign : Signum
  Stromtabelle Entladen : Lookup_n-D  NumberOfTableDimensions=1  BreakpointsForDimension1=[SpdRtrMecMin SpdRtrMecMin+SpdRtrMecMin*.1 SpdRtrMecMax]  Table=[0 1 1]  RndMeth=Simplest  InputSameDT=on
  Stromtabelle Laden : Lookup_n-D  NumberOfTableDimensions=1  BreakpointsForDimension1=[0 SpdRtrMecMax-SpdRtrMecMax*.1 SpdRtrMecMax]  Table=[1 1 0]  RndMeth=Simplest  InputSameDT=on
  Winkeltabelle Entaden : Lookup_n-D  NumberOfTableDimensions=1  BreakpointsForDimension1=[0 1]  Table=[-pi/4 -pi/4]  RndMeth=Simplest  InputSameDT=on
  Winkeltabelle Laden : Lookup_n-D  NumberOfTableDimensions=1  BreakpointsForDimension1=[0 1]  Table=[pi/4 pi/4 ]  RndMeth=Simplest  InputSameDT=on
  AgDeltaCurRtrDqSp : Outport
  AmpCurRtrDqSp : Outport  Port=2
  wires:
  PwrDcCnvrSp/1 -> Regler_Amplitude/1(Soll)
  IDcCnvrMeas/1 -> Product/1
  UDcMeas/1 -> Product/2
  Product/1 -> Regler_Amplitude/2(Ist)
  Regler_Amplitude/2(fehler) -> Sign/1
  SpdRtrMecMeas/1 -> Stromtabelle Laden/1, Stromtabelle Entladen/1, Winkeltabelle Laden/1, Winkeltabelle Entaden/1
  Sign/1 -> Compare To Zero/1, Compare To Zero1/1
  Winkeltabelle Laden/1 -> Product1/1
  Winkeltabelle Entaden/1 -> Product2/1
  Stromtabelle Laden/1 -> Product3/1
  Stromtabelle Entladen/1 -> Product4/1
  Compare To Zero/1 -> Product3/2, Product1/2
  Compare To Zero1/1 -> Product4/2, Product2/2
  Product1/1 -> Add/1
  Product2/1 -> Add/2
  Add/1 -> AgDeltaCurRtrDqSp/1
  Product3/1 -> Add1/1
  Product4/1 -> Add1/2
  Add1/1 -> Product5/2
  Regler_Amplitude/1(Stell) -> Product5/1
  Product5/1 -> Saturation/1
  Saturation/1 -> AmpCurRtrDqSp/1

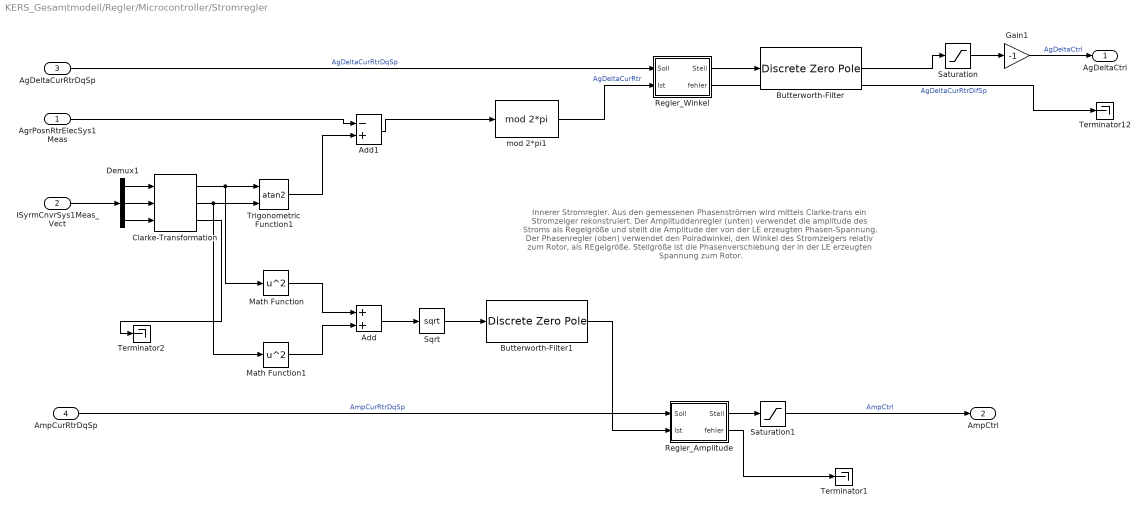
== system KERS_Gesamtmodell/Regler/Microcontroller/Stromregler ==
  note: Innerer Stromregler. Aus den gemessenen Phasenströmen wird mittels
      | Clarke-trans ein Stromzeiger rekonstruiert. Der Amplituddenregler (unten)
      | verwendet die amplitude des Stroms als Regelgröße und stellt die Amplitude
      | der von der LE erzeugten Phasen-Spannung.
      | Der Phasenregler (oben) verwendet den Polradwinkel, den Winkel des
      | Stromzeigers relativ zum Rotor, als REgelgröße. Stellgröße ist die
      | Phasenverschiebung der in der LE erzeugten Spannung zum Rotor.
  AgrPosnRtrElecSys1Meas : Inport
  ISyrmCnvrSys1Meas_Vect : Inport  Port=2
  AgDeltaCurRtrDqSp : Inport  Port=3
  AmpCurRtrDqSp : Inport  Port=4
  Add : Sum
  Add1 : Sum  Inputs=-+
  Butterworth-Filter : DiscreteZeroPole  Zeros=CoeffFiltZ  Poles=CoeffFiltP  Gain=CoeffFiltK  SampleTime=-1
  Butterworth-Filter1 : DiscreteZeroPole  Zeros=CoeffFiltZ  Poles=CoeffFiltP  Gain=CoeffFiltK  SampleTime=-1
  Clarke-Transformation : KERS_SystemModel_lib/Transformationen/Clarke-Transformation  SystemSampleTime=-1
  Demux1 : Demux  Outputs=3
  Gain1 : Gain  Gain=-1
  Math Function : Math  Operator=square  SaturateOnIntegerOverflow=on
  Math Function1 : Math  Operator=square  SaturateOnIntegerOverflow=on
  Regler_Amplitude : Subsystem
  Regler_Winkel : Subsystem
  Saturation : Saturate  UpperLimit=pi  LowerLimit=-pi
  Saturation1 : Saturate  UpperLimit=1  LowerLimit=0
  Sqrt : Sqrt  SaturateOnIntegerOverflow=on
  Terminator1 : Terminator
  Terminator12 : Terminator
  Terminator2 : Terminator
  Trigonometric Function1 : Trigonometry  Operator=atan2
  mod 2*pi1 : KERS_SystemModel_lib/Transformationen/mod 2*pi  SystemSampleTime=-1  tau=2*pi
  AgDeltaCtrl : Outport
  AmpCtrl : Outport  Port=2
  wires:
  Demux1/1 -> Clarke-Transformation/1
  Demux1/2 -> Clarke-Transformation/2
  Demux1/3 -> Clarke-Transformation/3
  ISyrmCnvrSys1Meas_Vect/1 -> Demux1/1
  AgrPosnRtrElecSys1Meas/1 -> Add1/1
  Regler_Winkel/1(Stell) -> Butterworth-Filter/1
  Add1/1 -> mod 2*pi1/1
  Trigonometric Function1/1 -> Add1/2
  Regler_Winkel/2(fehler) -> Terminator12/1  "AgDeltaCurRtrDifSp"
  AgDeltaCurRtrDqSp/1 -> Regler_Winkel/1(Soll)  "AgDeltaCurRtrDqSp"
  mod 2*pi1/1 -> Regler_Winkel/2(Ist)  "AgDeltaCurRtr"
  Clarke-Transformation/1 -> Trigonometric Function1/1, Math Function/1
  Clarke-Transformation/2 -> Trigonometric Function1/2, Math Function1/1
  Saturation/1 -> Gain1/1
  Gain1/1 -> AgDeltaCtrl/1  "AgDeltaCtrl"
  Regler_Amplitude/1(Stell) -> Saturation1/1
  AmpCurRtrDqSp/1 -> Regler_Amplitude/1(Soll)  "AmpCurRtrDqSp"
  Math Function/1 -> Add/1
  Math Function1/1 -> Add/2
  Add/1 -> Sqrt/1
  Sqrt/1 -> Butterworth-Filter1/1
  Saturation1/1 -> AmpCtrl/1  "AmpCtrl"
  Butterworth-Filter1/1 -> Regler_Amplitude/2(Ist)
  Regler_Amplitude/2(fehler) -> Terminator1/1
  Clarke-Transformation/3 -> Terminator2/1
  Butterworth-Filter/1 -> Saturation/1

== system KERS_Gesamtmodell/Regler/FPGA/Ansteuerung LE/Triggered Subsystem ==
  In1 : Inport
  Trigger : TriggerPort  TriggerType=falling
  Out1 : Outport
  wires:
  In1/1 -> Out1/1

== system KERS_Gesamtmodell/Regler/Microcontroller/Leistungsregler (INAKTIV)/Regler_Amplitude ==
  Soll : Inport
  Ist : Inport  Port=2
  Add1 : Sum  Inputs=+-
  Add2 : Sum
  Discrete-Time Integrator : DiscreteIntegrator  SampleTime=-1  ICPrevOutput=DiscIntNeverNeededParam  ICPrevScaledInput=DiscIntNeverNeededParam
  Gain : Gain  Gain=0.0001
  Gain1 : Gain  Gain=0.2
  Stell : Outport
  fehler : Outport  Port=2
  wires:
  Discrete-Time Integrator/1 -> Gain1/1
  Gain1/1 -> Add2/2
  Gain/1 -> Add2/1
  Add2/1 -> Stell/1
  Add1/1 -> fehler/1, Discrete-Time Integrator/1, Gain/1
  Ist/1 -> Add1/2
  Soll/1 -> Add1/1

== system KERS_Gesamtmodell/Regler/Microcontroller/Stromregler/Regler_Amplitude ==
  Soll : Inport
  Ist : Inport  Port=2
  Add1 : Sum  Inputs=+-
  Add2 : Sum
  Discrete-Time Integrator : DiscreteIntegrator  InitialCondition=1  SampleTime=-1  ICPrevOutput=DiscIntNeverNeededParam  ICPrevScaledInput=DiscIntNeverNeededParam
  Gain : Gain  Gain=0.000000001
  Gain2 : Gain  Gain=0.002
  Stell : Outport
  fehler : Outport  Port=2
  wires:
  Discrete-Time Integrator/1 -> Add2/2
  Gain/1 -> Add2/1
  Add2/1 -> Stell/1
  Add1/1 -> fehler/1, Gain2/1, Gain/1
  Ist/1 -> Add1/2
  Soll/1 -> Add1/1
  Gain2/1 -> Discrete-Time Integrator/1

== system KERS_Gesamtmodell/Regler/Microcontroller/Stromregler/Regler_Winkel ==
  Soll : Inport
  Ist : Inport  Port=2
  Add1 : Sum  Inputs=+-
  Add2 : Sum
  Discrete-Time Integrator : DiscreteIntegrator  SampleTime=-1  ICPrevOutput=DiscIntNeverNeededParam  ICPrevScaledInput=DiscIntNeverNeededParam
  Gain : Gain  Gain=0000.0001
  Gain1 : Gain  Gain=10
  Gain2 : Gain  Gain=-1
  Stell : Outport
  fehler : Outport  Port=2
  wires:
  Soll/1 -> Add1/1
  Ist/1 -> Add1/2
  Add1/1 -> Gain/1, fehler/1, Discrete-Time Integrator/1
  Add2/1 -> Gain2/1
  Gain/1 -> Add2/1
  Gain1/1 -> Add2/2
  Discrete-Time Integrator/1 -> Gain1/1
  Gain2/1 -> Stell/1
